simulink model "snrtest"  (R2014a)
settings: Solver=ode3  StartTime=0.0  StopTime=20  FixedStep=1/44100  RelTol=1e-3
values from neighbouring files (symbols this model uses):
  freq = 1000    [snrtestscript.m]
libraries: dspsrcs4 x1, dspsnks4 x1
settings Model: Creator=Administratör  LastModifiedBy=Administratör
settings OptimizationCC: InlineParams=on  InlineInvariantSignals=on  EfficientFloat2IntCast=on  SimCompilerOptimization=On

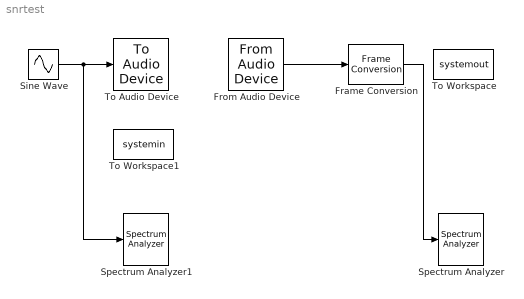
== system snrtest ==
  Frame Conversion : FrameConversion  OutFrame=Sample-based
  From Audio Device : dspsrcs4/From Audio Device  deviceName=Default  numChannels=1  sampleRate=44100  deviceDatatype=24-bit integer  autoBufferSize=off  bufferSize=256  queueDuration=1  frameSize=1  outputDatatype=double  defaultInputChannelMapping=on  inputChannelMapping=1:2
  Sine Wave : Sin  Frequency=2*pi*freq
  Spectrum Analyzer : SpectrumAnalyzer
  Spectrum Analyzer1 : SpectrumAnalyzer
  To Audio Device : dspsnks4/To Audio Device  deviceName=Default  inheritSampleRate=off  sampleRate=44100  deviceDatatype=Determine from input data type  autoBufferSize=off  bufferSize=256  queueDuration=1  defaultOutputChannelMapping=on  outputChannelMapping=1:2
  To Workspace : ToWorkspace  VariableName=systemout  SaveFormat=Structure With Time  SampleTime=-1
  To Workspace1 : ToWorkspace  VariableName=systemin  SaveFormat=Structure With Time  SampleTime=-1
  wires:
  Sine Wave/1 -> Spectrum Analyzer1/1, To Audio Device/1
  From Audio Device/1 -> Frame Conversion/1
  Frame Conversion/1 -> Spectrum Analyzer/1
